simulink model "mainNewTraj"  (R2019b)
settings: Solver=VariableStepAuto  StartTime=0.0  StopTime=0.3  FixedStep=2e-4  RelTol=1e-3
values from neighbouring files (symbols this model uses):
  A1 = 8    [initSim.m]
  A2 = 5    [initSim.m]
  A3 = 3    [initSim.m]
  accCoef = x(1) + accCoef    [accJerkSnapFFtuning.m]    (also in initSim.m = sum(m))
  jerkCoef = x(2) + jerkCoef    [accJerkSnapFFtuning.m]    (also in initSim.m = sum(m) * tau)
  snapCoef = x(3) + snapCoef    [accJerkSnapFFtuning.m]    (also in initSim.m = sum(m) * ( 1/wn.^2 + 0.5 * tau.^2))
  Ts = 1/fs    [discretizeControllerWithFrequencyPrewarping.m]    (also in initSim.m = 0.0002; noncausalFiltering.m = noncausalFilter.Ts)
undefined symbols (not defined in the file or in its folder): DiscIntNeverNeededParam
libraries: cstblocks x3, simulink x1, model_controller x1
settings Model: Creator=Dai Luyao  LastModifiedBy=MyPrincess
settings DataIOCC: ReturnWorkspaceOutputs=off
settings DebuggingCC: ArithmeticOperatorsInVariantConditions=warning
settings SFSimCC: SimUseLocalCustomCode=off  CustomCodeUndefinedFunction=UseInterfaceOnly
settings RTWCC: RTWUseLocalCustomCode=off
settings CodeAppCC: StateflowObjectComments=on

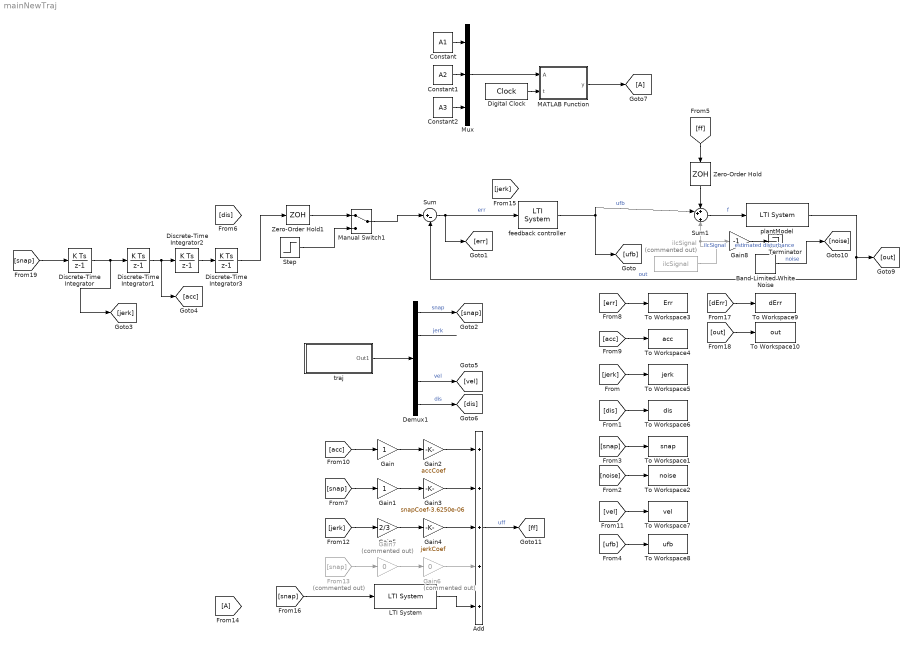
== system mainNewTraj ==
  Add : Sum  Inputs=+++++
  Band-Limited White Noise : simulink/Sources/Band-Limited White Noise  Cov=noisePower  Ts=Ts  seed=[2331]
  Constant : Constant  Value=A1
  Constant1 : Constant  Value=A2
  Constant2 : Constant  Value=A3
  Demux1 : Demux  Outputs=5
  Digital Clock : DigitalClock  SampleTime=Ts
  Discrete-Time Integrator{,1..3} (4 alike) : DiscreteIntegrator  SampleTime=-1  ICPrevOutput=DiscIntNeverNeededParam  ICPrevScaledInput=DiscIntNeverNeededParam
  From13 : From  Commented=on  GotoTag=snap
  Gain : Gain
  Gain1 : Gain
  Gain2 : Gain  Gain=accCoef
  Gain3 : Gain  Gain=snapCoef-3.6250e-06
  Gain4 : Gain  Gain=jerkCoef
  Gain5 : Gain  Gain=2/3
  Gain6 : Gain  Commented=on  Gain=0
  Gain7 : Gain  Commented=on  Gain=0
  Gain8 : Gain  Gain=-1
  LTI System : cstblocks/LTI System  sys=GStableNew  IC=[]
  MATLAB Function : MATLAB Function  TreatAsAtomicUnit=on
  Manual Switch1 : ManualSwitch
  Mux : Mux  Inputs=3
  Step : Step  Time=0  After=30e-6  SampleTime=0
  Sum : Sum  Inputs=|+-
  Sum1 : Sum  Inputs=++|+
  Terminator : Terminator
  To Workspace1 : ToWorkspace  VariableName=snap  SaveFormat=Structure With Time  SampleTime=Ts
  To Workspace10 : ToWorkspace  VariableName=out  SaveFormat=Structure With Time  SampleTime=Ts
  To Workspace2 : ToWorkspace  VariableName=noise  SaveFormat=Structure With Time  SampleTime=Ts
  To Workspace3 : ToWorkspace  VariableName=Err  SaveFormat=Structure With Time  SampleTime=Ts
  To Workspace4 : ToWorkspace  VariableName=acc  SaveFormat=Structure With Time  SampleTime=Ts
  To Workspace5 : ToWorkspace  VariableName=jerk  SaveFormat=Structure With Time  SampleTime=Ts
  To Workspace6 : ToWorkspace  VariableName=dis  SaveFormat=Structure With Time  SampleTime=Ts
  To Workspace7 : ToWorkspace  VariableName=vel  SaveFormat=Structure With Time  SampleTime=Ts
  To Workspace8 : ToWorkspace  VariableName=ufb  SaveFormat=Structure With Time  SampleTime=Ts
  To Workspace9 : ToWorkspace  VariableName=dErr  SaveFormat=Structure With Time  SampleTime=Ts
  Zero-Order Hold : ZeroOrderHold  SampleTime=Ts
  Zero-Order Hold1 : ZeroOrderHold  SampleTime=Ts
  feedback controller : cstblocks/LTI System  sys=GcDis  IC=[]
  ilcSignal : FromWorkspace  Commented=on  VariableName=ilcSignal  SampleTime=Ts
  plantModel : cstblocks/LTI System  sys=GpDis  IC=[]
  traj : Subsystem  BlockChoice=4th order traj
      link override 2nd order traj: x=0.6  v=0.25  a=10
      link override 3rd order traj: j=trajParameters.jerk  v=trajParameters.vel  x=trajParameters.dis  a=trajParameters.acc
      link override 4th order traj: a=10  v=0.25  x=0.04  j=800  d=64000  Ts=0  t0=0.02
      link override step: vf=1e-6
      settings: AttributesFormatString=%<BlockChoice>  TemplateBlock=model_controller/Profile Generators/traj  MemberBlocks=2th order traj,3rd order traj,4th order traj,step
  wires:
  Sum/1 -> feedback controller/1, [err]  "err"
  Demux1/1 -> [snap]  "snap"
  Demux1/2 -> ?  "jerk"
  Demux1/4 -> [vel]  "vel"
  Demux1/5 -> [dis]  "dis"
  [acc] -> To Workspace4/1
  [acc] -> Gain/1
  [jerk] -> To Workspace5/1
  [dis] -> To Workspace6/1
  [err] -> To Workspace3/1
  [noise] -> To Workspace2/1
  [ff] -> Zero-Order Hold/1
  [snap] -> To Workspace1/1
  [snap] -> Gain1/1
  Gain/1 -> Gain2/1
  Gain1/1 -> Gain3/1
  Add/1 -> [ff]  "uff"
  Gain2/1 -> Add/1
  Gain3/1 -> Add/2
  [vel] -> To Workspace7/1
  Gain4/1 -> Add/3
  [jerk] -> Gain5/1
  Gain5/1 -> Gain4/1
  Gain7/1 -> Gain6/1
  From13/1 -> Gain7/1
  Gain6/1 -> Add/4
  plantModel/1 -> [out], Sum/2  "out"
  traj/1(Out1) -> Demux1/1
  feedback controller/1 -> [ufb], Sum1/2  "ufb"
  Sum1/1 -> plantModel/1  "f"
  [ufb] -> To Workspace8/1
  Zero-Order Hold/1 -> Sum1/1
  Step/1 -> Manual Switch1/2
  Zero-Order Hold1/1 -> Manual Switch1/1
  Band-Limited White Noise/1 -> [noise]  "noise"
  [dErr] -> To Workspace9/1
  [out] -> To Workspace10/1
  ilcSignal/1 -> Gain8/1, Sum1/3  "ilcSignal"
  Constant/1 -> Mux/1
  Constant1/1 -> Mux/2
  Constant2/1 -> Mux/3
  Mux/1 -> MATLAB Function/1(A)
  Digital Clock/1 -> MATLAB Function/2(t)
  MATLAB Function/1(y) -> [A]
  Gain8/1 -> Terminator/1  "estimated disturbance"
  Manual Switch1/1 -> Sum/1
  [snap] -> LTI System/1
  [snap] -> Discrete-Time Integrator/1
  Discrete-Time Integrator/1 -> [jerk], Discrete-Time Integrator1/1
  Discrete-Time Integrator1/1 -> [acc], Discrete-Time Integrator2/1
  Discrete-Time Integrator2/1 -> Discrete-Time Integrator3/1
  Discrete-Time Integrator3/1 -> Zero-Order Hold1/1
  LTI System/1 -> Add/5

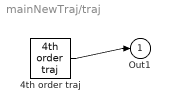
== system mainNewTraj/traj ==
  4th order traj : model_controller/Profile Generators/4th order traj  t0=0.02  x=0.04  v=0.25  a=10  j=800  d=64000  Ts=0
  Out1 : Outport
  wires:
  4th order traj/1 -> Out1/1

== matlab function mainNewTraj/MATLAB Function ==
  data: A input; y output; t input
function y = fcn(A,t)
A1 = A(1);
A2 = A(2);
A3 = A(3);
f1 = 6;
f2 = 30;
f3 = 300;
w1 = 2 * pi * f1; phase1 = pi / 6;
w2 = 2 * pi * f2; phase2 = pi / 3;
w3 = 2 * pi * f3; phase3 = pi / 4;
y = A1 * sin(w1*t + phase1) + A2 * sin(w2*t + phase2) + A3 * sin(w3*t + phase3);
